simulink model "LinearDynamic"  (R2020b)
settings: Solver=VariableStepAuto  StartTime=0.0  StopTime=25  RelTol=1e-3
values from neighbouring files (symbols this model uses):
  l = 0.06    [VehicleModelDictionary.sldd]    (also in VehicleParameters.m; VehicleParametersDictionary.sldd)
  ltiSys = ss(ltiSys.A, ltiSys.B, C, D)    [ControllerDesign.m]    (also in LinearAnalysis.m = ss(A, B, C, D); VehicleModelDictionary.sldd = 4.0 2.0
                22.0
                
              )
undefined symbols (not defined in the file or in its folder): accel, gyro
libraries: simulink x2
Description:
  | Entorno de simulación lineal del vehículo
settings Model: Creator=Gonzalo Fernández  LastModifiedBy=Gonzalo Fernández

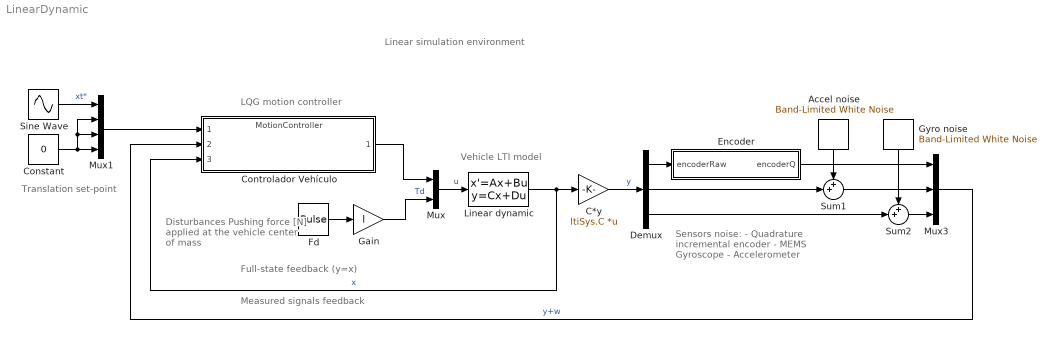
== system LinearDynamic ==
  note: Sensors noise:
      | - Quadrature incremental encoder
      | - MEMS Gyroscope
      | - Accelerometer
  note: Disturbances
      | Pushing force [N] applied at
      | the vehicle center of mass
  note: LQG motion controller
  note: Vehicle LTI model
  note: Translation set-point
  note: Measured signals feedback
  note: Full-state feedback (y=x)
  note: Linear simulation environment
  Accel noise : simulink/Sources/Band-Limited White Noise  Cov=(accel.RNoiseDensity)^2  Ts=1/accel.Fs  seed=[23341]
  C*y : Gain  Gain=ltiSys.C  Multiplication=Matrix(K*u)
  Constant : Constant  Value=0
  Controlador Vehículo : ModelReference  ModelNameDialog=MotionController.slx  SimulationMode=Normal  ModelReferenceVersion=1.31
  Demux : Demux  Outputs=3
  Encoder : Subsystem
  Fd : DiscretePulseGenerator  PulseType=Time based  Amplitude=0  Period=10  PulseWidth=5
  Gain : Gain  Gain=l
  Gyro noise : simulink/Sources/Band-Limited White Noise  Cov=(gyro.RNoiseDensity*pi/180)^2  Ts=1/gyro.Fs  seed=[23341]
  Linear dynamic : StateSpace  A=ltiSys.A  B=ltiSys.B  C=eye(4)  D=|  InitialCondition=[0; deg2rad(0); 0; 0]
      | [0, 0;
      | 0, 0; 0, 0; 0, 0]
  Mux : Mux  Inputs=2
  Mux1 : Mux
  Mux3 : Mux  Inputs=3
  Sine Wave : Sin  Amplitude=0.5  Frequency=2*pi/15  SampleTime=0
  Sum1 : Sum  Inputs=++|
  Sum2 : Sum  Inputs=++|
  wires:
  Mux/1 -> Linear dynamic/1  "u"
  Fd/1 -> Gain/1
  Linear dynamic/1 -> Controlador Vehículo/3, C*y/1  "x"
  Controlador Vehículo/1 -> Mux/1
  Mux1/1 -> Controlador Vehículo/1
  Constant/1 -> Mux1/2, Mux1/3, Mux1/4
  Sine Wave/1 -> Mux1/1  "xt*"
  Gain/1 -> Mux/2  "Td"
  C*y/1 -> Demux/1  "y"
  Mux3/1 -> Controlador Vehículo/2  "y+w"
  Accel noise/1 -> Sum1/1
  Sum1/1 -> Mux3/2
  Encoder/1(encoderQ) -> Mux3/1
  Demux/3 -> Sum2/2
  Demux/1 -> Encoder/1(encoderRaw)
  Sum2/1 -> Mux3/3
  Demux/2 -> Sum1/2
  Gyro noise/1 -> Sum2/1

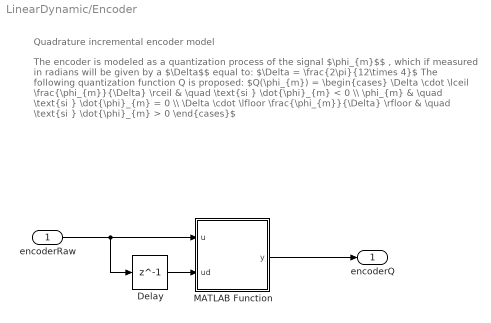
== system LinearDynamic/Encoder ==
  note: Quadrature incremental encoder model
  note: The encoder is modeled as a quantization process of the signal $\phi_{m}$$ , which if measured in radians will be given by a $\Delta$$ equal to:
      | $\Delta = \frac{2\pi}{12\times 4}$
      | The following quantization function Q is proposed:
      |
      | $Q(\phi_{m}) = \begin{cases} \Delta \cdot \lceil \frac{\phi_{m}}{\Delta} \rceil & \quad \text{si } \dot{\phi}_{m} < 0 \\ \phi_{m} & \quad \text{si } \dot{\phi}_{m} = 0 \\ \Delta \cdot \lfloor \frac{\phi_{m}}{\Delta} \rfloor & \quad \text{si } \dot{\phi}_{m} > 0 \end{cases}$
  encoderRaw : Inport
  Delay : Delay  DelayLength=1
  MATLAB Function : MATLAB Function  TreatAsAtomicUnit=on
  encoderQ : Outport
  wires:
  Delay/1 -> MATLAB Function/2(ud)
  encoderRaw/1 -> MATLAB Function/1(u), Delay/1
  MATLAB Function/1(y) -> encoderQ/1

== matlab function LinearDynamic/Encoder/MATLAB Function ==
  data: u input; y output; ud input; QuadratureEncoder parameter
function y = Q(u, ud, QuadratureEncoder)
delta = 2*pi/(QuadratureEncoder.PPR*QuadratureEncoder.ResolutionMult);
y = u/delta;
diff = u - ud;
if diff < 0
    y = ceil(y);
elseif diff > 0
    y = floor(y);
end
y = y*delta;
